simulink model "WaterTanks_10_Tanks_Model"  (Simulink 8.1)
settings: Solver=ode3  StartTime=0.0  StopTime=180.0  FixedStep=0.001  RelTol=1e-3
InitFcn:
  | initparametersDACADC
undefined symbols (not defined in the file): Ad, Bd, Cd, Dd, x0
libraries: GisooLib x21
settings Model: Creator=behdad  LastModifiedBy=behdad

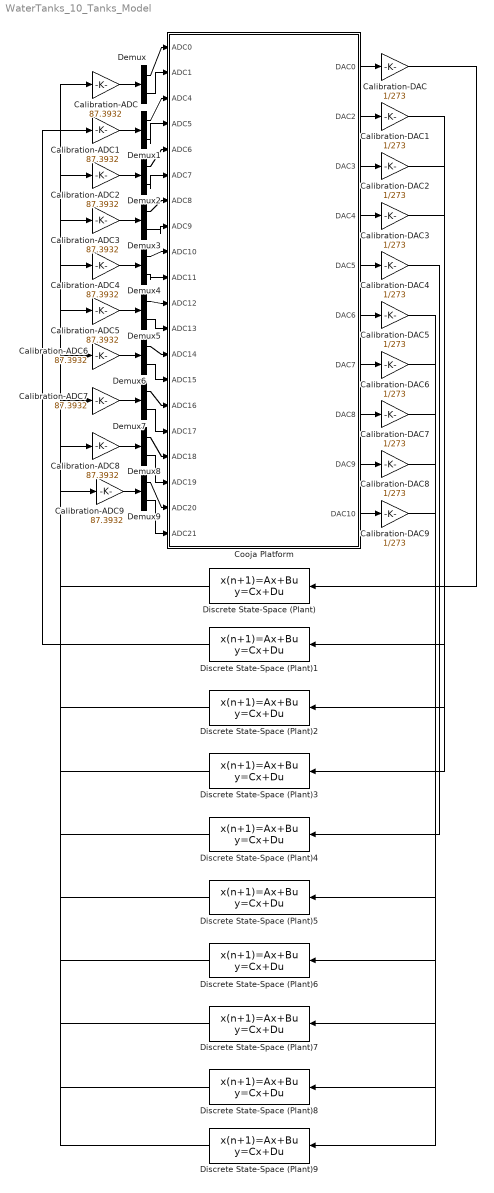
== system WaterTanks_10_Tanks_Model ==
  Calibration-ADC{,1..9} (10 alike) : Gain  Gain=87.3932
  Calibration-DAC{,1..9} (10 alike) : Gain  Gain=1/273
  Cooja Platform : Subsystem  AncestorBlock=GisooLib/Gisoo Platform  TreatAsAtomicUnit=on
  Demux{,1..9} (10 alike) : Demux  Outputs=2
  Discrete State-Space (Plant){,1..9} (10 alike) : DiscreteStateSpace  A=Ad  B=Bd  C=Cd  D=Dd  X0=x0  SampleTime=-1
  wires:
  Discrete State-Space (Plant)/1 -> Calibration-ADC/1
  Calibration-ADC/1 -> Demux/1
  Demux/1 -> Cooja Platform/1(ADC0)
  Demux/2 -> Cooja Platform/2(ADC1)
  Calibration-DAC/1 -> Discrete State-Space (Plant)/1
  Cooja Platform/1(DAC0) -> Calibration-DAC/1
  Cooja Platform/2(DAC2) -> Calibration-DAC1/1
  Cooja Platform/3(DAC3) -> Calibration-DAC2/1
  Cooja Platform/4(DAC4) -> Calibration-DAC3/1
  Cooja Platform/5(DAC5) -> Calibration-DAC4/1
  Cooja Platform/6(DAC6) -> Calibration-DAC5/1
  Cooja Platform/7(DAC7) -> Calibration-DAC6/1
  Cooja Platform/8(DAC8) -> Calibration-DAC7/1
  Cooja Platform/9(DAC9) -> Calibration-DAC8/1
  Cooja Platform/10(DAC10) -> Calibration-DAC9/1
  Calibration-DAC1/1 -> Discrete State-Space (Plant)1/1
  Calibration-DAC2/1 -> Discrete State-Space (Plant)2/1
  Calibration-DAC3/1 -> Discrete State-Space (Plant)3/1
  Calibration-DAC4/1 -> Discrete State-Space (Plant)4/1
  Calibration-DAC5/1 -> Discrete State-Space (Plant)5/1
  Calibration-DAC6/1 -> Discrete State-Space (Plant)6/1
  Calibration-DAC7/1 -> Discrete State-Space (Plant)7/1
  Calibration-DAC8/1 -> Discrete State-Space (Plant)8/1
  Calibration-DAC9/1 -> Discrete State-Space (Plant)9/1
  Calibration-ADC1/1 -> Demux1/1
  Calibration-ADC2/1 -> Demux2/1
  Calibration-ADC3/1 -> Demux3/1
  Calibration-ADC4/1 -> Demux4/1
  Calibration-ADC5/1 -> Demux5/1
  Calibration-ADC6/1 -> Demux6/1
  Calibration-ADC7/1 -> Demux7/1
  Demux1/1 -> Cooja Platform/3(ADC4)
  Demux1/2 -> Cooja Platform/4(ADC5)
  Demux2/1 -> Cooja Platform/5(ADC6)
  Demux2/2 -> Cooja Platform/6(ADC7)
  Demux3/1 -> Cooja Platform/7(ADC8)
  Demux3/2 -> Cooja Platform/8(ADC9)
  Demux4/1 -> Cooja Platform/9(ADC10)
  Demux4/2 -> Cooja Platform/10(ADC11)
  Demux5/1 -> Cooja Platform/11(ADC12)
  Demux5/2 -> Cooja Platform/12(ADC13)
  Demux6/1 -> Cooja Platform/13(ADC14)
  Demux6/2 -> Cooja Platform/14(ADC15)
  Demux7/1 -> Cooja Platform/15(ADC16)
  Demux7/2 -> Cooja Platform/16(ADC17)
  Demux8/1 -> Cooja Platform/17(ADC18)
  Demux8/2 -> Cooja Platform/18(ADC19)
  Demux9/1 -> Cooja Platform/19(ADC20)
  Demux9/2 -> Cooja Platform/20(ADC21)
  Calibration-ADC9/1 -> Demux9/1
  Calibration-ADC8/1 -> Demux8/1
  Discrete State-Space (Plant)1/1 -> Calibration-ADC1/1
  Discrete State-Space (Plant)2/1 -> Calibration-ADC2/1
  Discrete State-Space (Plant)3/1 -> Calibration-ADC3/1
  Discrete State-Space (Plant)4/1 -> Calibration-ADC4/1
  Discrete State-Space (Plant)5/1 -> Calibration-ADC5/1
  Discrete State-Space (Plant)6/1 -> Calibration-ADC6/1
  Discrete State-Space (Plant)7/1 -> Calibration-ADC7/1
  Discrete State-Space (Plant)8/1 -> Calibration-ADC8/1
  Discrete State-Space (Plant)9/1 -> Calibration-ADC9/1

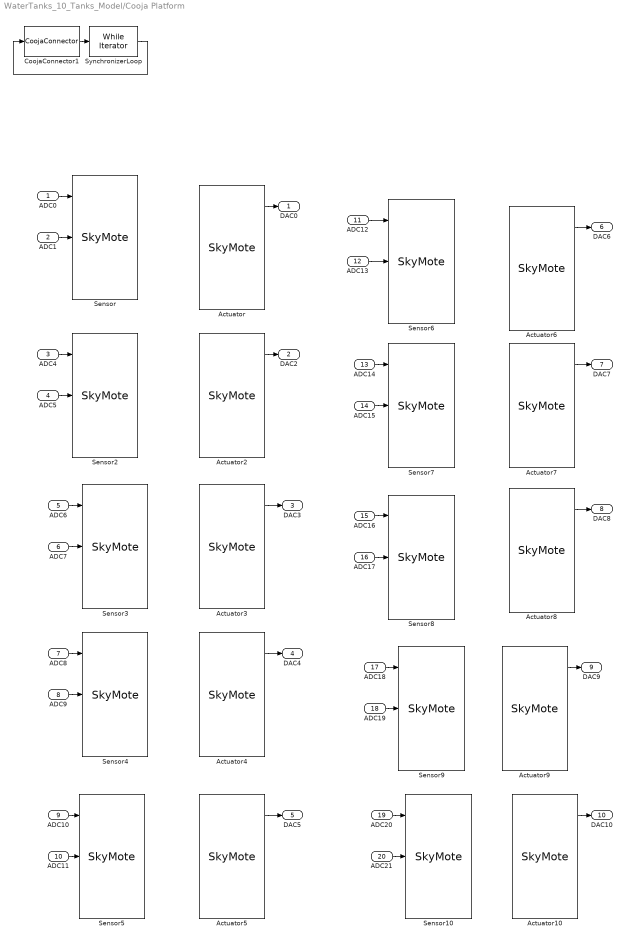
== system WaterTanks_10_Tanks_Model/Cooja Platform ==
  ADC0 : Inport
  ADC1 : Inport  Port=2
  ADC4 : Inport  Port=3
  ADC5 : Inport  Port=4
  ADC6 : Inport  Port=5
  ADC7 : Inport  Port=6
  ADC8 : Inport  Port=7
  ADC9 : Inport  Port=8
  ADC10 : Inport  Port=9
  ADC11 : Inport  Port=10
  ADC12 : Inport  Port=11
  ADC13 : Inport  Port=12
  ADC14 : Inport  Port=13
  ADC15 : Inport  Port=14
  ADC16 : Inport  Port=15
  ADC17 : Inport  Port=16
  ADC18 : Inport  Port=17
  ADC19 : Inport  Port=18
  ADC20 : Inport  Port=19
  ADC21 : Inport  Port=20
  Actuator : GisooLib/SkyMote  moteID=21  PacketType=6
  Actuator10 : GisooLib/SkyMote  moteID=30  PacketType=6
  Actuator2 : GisooLib/SkyMote  moteID=22  PacketType=6
  Actuator3 : GisooLib/SkyMote  moteID=23  PacketType=6
  Actuator4 : GisooLib/SkyMote  moteID=24  PacketType=6
  Actuator5 : GisooLib/SkyMote  moteID=25  PacketType=6
  Actuator6 : GisooLib/SkyMote  moteID=26  PacketType=6
  Actuator7 : GisooLib/SkyMote  moteID=27  PacketType=6
  Actuator8 : GisooLib/SkyMote  moteID=28  PacketType=6
  Actuator9 : GisooLib/SkyMote  moteID=29  PacketType=6
  CoojaConnector1 : GisooLib/Cooja Platform/CoojaConnector
      link override "Check that we don't loop forever, if Cooja never answers": const=900000
  Sensor : GisooLib/SkyMote  moteID=1  PacketType=6
  Sensor10 : GisooLib/SkyMote  moteID=10  PacketType=6
  Sensor2 : GisooLib/SkyMote  moteID=2  PacketType=6
  Sensor3 : GisooLib/SkyMote  moteID=3  PacketType=6
  Sensor4 : GisooLib/SkyMote  moteID=4  PacketType=6
  Sensor5 : GisooLib/SkyMote  moteID=5  PacketType=6
  Sensor6 : GisooLib/SkyMote  moteID=6  PacketType=6
  Sensor7 : GisooLib/SkyMote  moteID=7  PacketType=6
  Sensor8 : GisooLib/SkyMote  moteID=8  PacketType=6
  Sensor9 : GisooLib/SkyMote  moteID=9  PacketType=6
  SynchronizerLoop : WhileIterator  MaxIters=-1  WhileBlockType=do-while  ShowIterationPort=on
  DAC0 : Outport
  DAC2 : Outport  Port=2
  DAC3 : Outport  Port=3
  DAC4 : Outport  Port=4
  DAC5 : Outport  Port=5
  DAC6 : Outport  Port=6
  DAC7 : Outport  Port=7
  DAC8 : Outport  Port=8
  DAC9 : Outport  Port=9
  DAC10 : Outport  Port=10
  wires:
  Actuator/1 -> DAC0/1
  ADC0/1 -> Sensor/1
  ADC1/1 -> Sensor/2
  Actuator2/1 -> DAC2/1
  ADC4/1 -> Sensor2/1
  ADC5/1 -> Sensor2/2
  Actuator3/1 -> DAC3/1
  ADC6/1 -> Sensor3/1
  ADC7/1 -> Sensor3/2
  Actuator4/1 -> DAC4/1
  ADC8/1 -> Sensor4/1
  ADC9/1 -> Sensor4/2
  Actuator5/1 -> DAC5/1
  ADC10/1 -> Sensor5/1
  ADC11/1 -> Sensor5/2
  Actuator6/1 -> DAC6/1
  ADC12/1 -> Sensor6/1
  ADC13/1 -> Sensor6/2
  Actuator7/1 -> DAC7/1
  ADC14/1 -> Sensor7/1
  ADC15/1 -> Sensor7/2
  Actuator8/1 -> DAC8/1
  ADC16/1 -> Sensor8/1
  ADC17/1 -> Sensor8/2
  Actuator9/1 -> DAC9/1
  ADC18/1 -> Sensor9/1
  ADC19/1 -> Sensor9/2
  Actuator10/1 -> DAC10/1
  ADC20/1 -> Sensor10/1
  ADC21/1 -> Sensor10/2
  SynchronizerLoop/1 -> CoojaConnector1/1
  CoojaConnector1/1 -> SynchronizerLoop/1
